simulink model "gm_sampleModel1507_5_sub"  (R2023a)
settings: Solver=VariableStepAuto  StartTime=0.0  StopTime=10.0  RelTol=1e-3
libraries: simulink x3
settings Model: Creator=user1  LastModifiedBy=user1
settings OptimizationCC: BlockReduction=off  ConditionallyExecuteInputs=off
settings DebuggingCC: InheritedTsInSrcMsg=none

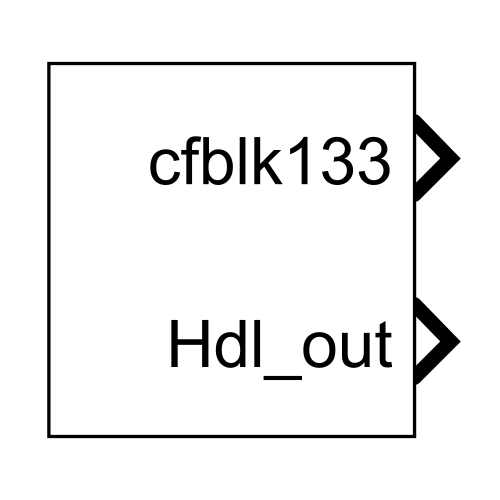
[thumbnail: Simulink's stored preview of the top-level diagram]
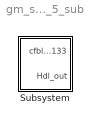
== system gm_sampleModel1507_5_sub ==
  Subsystem : Subsystem

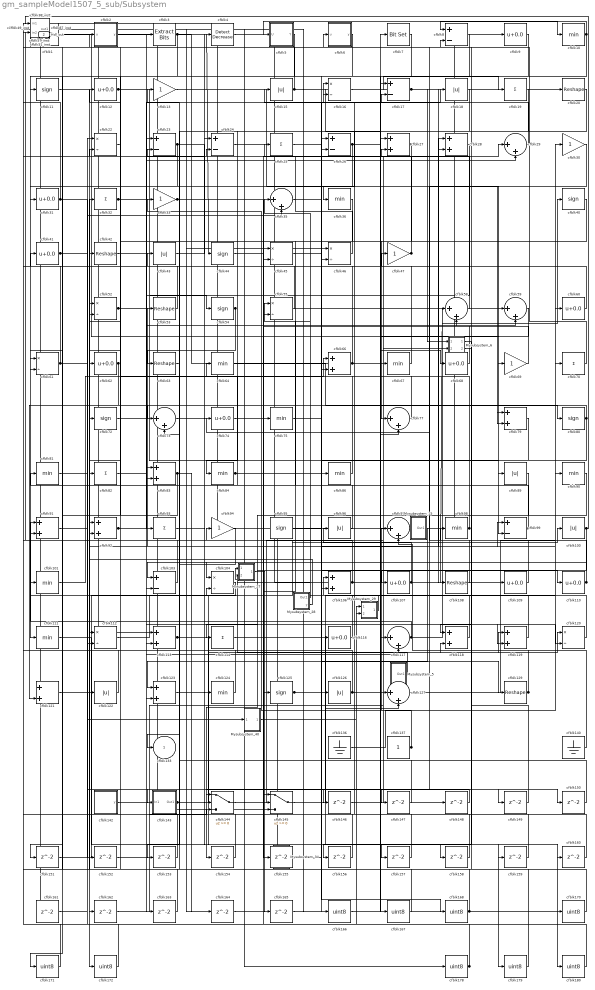
== system gm_sampleModel1507_5_sub/Subsystem ==
  Mysubsystem_15 : Subsystem
  Mysubsystem_27 : Subsystem
  Mysubsystem_28 : Subsystem
  Mysubsystem_29 : Subsystem
  Mysubsystem_34 : Subsystem
  Mysubsystem_40 : Subsystem
  Mysubsystem_5 : Subsystem
  Mysubsystem_6 : Subsystem
  cfblk1 : Logic  AllPortsSameDT=off  OutDataTypeStr=boolean
  cfblk{10,36,64,67,75,81,84,86,90,98,101,111,124} (13 alike) : MinMax  OutDataTypeStr=uint8
  cfblk{15,18,43,89,96,100,122,126} (8 alike) : Abs  OutDataTypeStr=uint8  SaturateOnIntegerOverflow=off
  cfblk102_inst : Subsystem
  cfblk{8,17,23..24,26,99,103} (7 alike) : Sum  Inputs=+-  OutDataTypeStr=uint8
  cfblk{16,22,45..46,52,55,61,104,112,120} (10 alike) : Product  Inputs=*/  OutDataTypeStr=uint8  RndMeth=Zero  SaturateOnIntegerOverflow=on
  cfblk{27..28,66,79,83,91..92,106,113,118..119,121,123} (13 alike) : Sum  OutDataTypeStr=uint8
  cfblk{9,12,31,41,60,62,68,74,107,109..110,116} (12 alike) : Bias  Bias=0.0  SaturateOnIntegerOverflow=off
  cfblk{20,42,53,63,108,129} (6 alike) : Reshape
  cfblk{11,40,44,54,72,80,95,125} (8 alike) : Signum
  cfblk{19,25,32,70,82,93,114} (7 alike) : Sum  Inputs=+  OutDataTypeStr=uint8
  cfblk{29,35,58..59,73,77,97,117,127} (9 alike) : Sum  Inputs=|++  OutDataTypeStr=uint8
  cfblk128_inst : Subsystem
  cfblk{13,30,33,47,69,94} (6 alike) : Gain  OutDataTypeStr=uint8
  cfblk136 : Ground
  cfblk137 : Constant  OutDataTypeStr=uint8  SampleTime=-1
  cfblk140 : Ground
  cfblk142 : Subsystem  mask(Counter Limited){uplimit=double(7), tsamp=double(-1)}
      mask prompts: uplimit "Simulink:masks:UpperLimit_MP"; tsamp "Simulink:masks:SampleTime_MP"
      mask help: Simulink:masks:CounterLimited_MD
      mask init:
      | nbits = double(8);
      | tsamp = double(-1);
      | uplimit = double(7);
  cfblk143 : Subsystem
  cfblk144 : Switch  OutDataTypeStr=uint8  SaturateOnIntegerOverflow=off  InputSameDT=off
  cfblk145 : Switch  OutDataTypeStr=uint8  SaturateOnIntegerOverflow=off  InputSameDT=off
  cfblk{146..165} (20 alike) : Delay  SampleTime=1
  cfblk{166..168,170..172,178..180} (9 alike) : DataTypeConversion  OutDataTypeStr=uint8  SaturateOnIntegerOverflow=off  RndMeth=Floor
  cfblk2 : Subsystem  mask(Compare To Zero){relop=<=, OutDataTypeStr=uint8, ZeroCross=on}
      mask prompts: relop "Simulink:masks:Operator_MP"; OutDataTypeStr "Simulink:masks:OutputDataType_MP"; ZeroCross "Simulink:masks:EnableZerocrossingDetection_MP"
      mask help: Simulink:masks:CompareToZero_MD
      mask init:
      | OutDataTypeStr = 'uint8';
      | ZeroCross = 'on';
      | blkName = 'sampleModel1507_5_sub/Subsystem/cfblk2';
      | relop = '<=';
      | setValue = 'fixdt(0, 8)';
      mask TypeOptions relop: == | ~= | < | <= | >= | >
      mask TypeOptions OutDataTypeStr: Simulink:masks:uint8 | Simulink:masks:boolean
      mask Callback ZeroCross: sl('zeroCrossEnable', gcbh);
      mask Display: disp([relop,' 0'])
  cfblk21_inst : Subsystem
  cfblk3 : simulink/Logic and Bit Operations/Extract Bits  bitsToExtract=Upper half  numBits=8  bitIdxRange=[0 7]  outScalingMode=Preserve fixed-point scaling
      settings: LibrarySourceBlock=|
      | hdlsllib/Logic and Bit
      | Operations/Extract Bits
  cfblk34_inst : Subsystem
  cfblk37_inst : Subsystem
  cfblk38_inst : Subsystem
  cfblk4 : simulink/Logic and Bit Operations/Detect Decrease  vinit=0.0  OutDataTypeStr=uint8
      settings: LibrarySourceBlock=|
      | hdlsllib/Logic and Bit
      | Operations/Detect
      | Decrease
  cfblk49_inst : Subsystem
  cfblk5 : Subsystem  mask(Detect Fall Nonpositive){vinit=double(0), InputProcessing=Elements as channels (sample based), OutDataTypeStr=uint8}
      mask prompts: vinit "Simulink:masks:InitialCondition_MP"; InputProcessing "Simulink:masks:InputProcessing_MP"; OutDataTypeStr "Simulink:masks:OutputDataType_MP"
      mask help: Simulink:masks:DetectFallNonpositive_MD
      mask init:
      | InputProcessing = 'Elements as channels (sample based)';
      | OutDataTypeStr = 'uint8';
      | vinit = double(0);
      mask TypeOptions InputProcessing: Simulink:masks:ColumnsAsChannelsFrameBased | Simulink:masks:ElementsAsChannelsSampleBased
      mask TypeOptions OutDataTypeStr: Simulink:masks:uint8 | Simulink:masks:boolean
      mask Display: fprintf('U <= 0\n&  NOT\nU/z <= 0')
  cfblk51_inst : Subsystem
  cfblk57_inst : Subsystem
  cfblk6 : Subsystem  mask(Compare To Zero){relop=<=, OutDataTypeStr=uint8, ZeroCross=on}
      mask prompts: relop "Simulink:masks:Operator_MP"; OutDataTypeStr "Simulink:masks:OutputDataType_MP"; ZeroCross "Simulink:masks:EnableZerocrossingDetection_MP"
      mask help: Simulink:masks:CompareToZero_MD
      mask init:
      | OutDataTypeStr = 'uint8';
      | ZeroCross = 'on';
      | blkName = 'sampleModel1507_5_sub/Subsystem/cfblk6';
      | relop = '<=';
      | setValue = 'fixdt(0, 8)';
      mask TypeOptions relop: == | ~= | < | <= | >= | >
      mask TypeOptions OutDataTypeStr: Simulink:masks:uint8 | Simulink:masks:boolean
      mask Callback ZeroCross: sl('zeroCrossEnable', gcbh);
      mask Display: disp([relop,' 0'])
  cfblk7 : simulink/Logic and Bit Operations/Bit Set  iBit=0
      settings: LibrarySourceBlock=|
      | hdlsllib/Logic and Bit
      | Operations/Bit Set
  cfblk87_inst : Subsystem
  cfblk133 : Outport  OutDataTypeStr=uint8  SampleTime=1  VectorParamsAs1DForOutWhenUnconnected=off
  Hdl_out : Outport  Port=2  OutDataTypeStr=uint8  SampleTime=1
  wires:
  Mysubsystem_15/1(Out1) -> cfblk123/1
  Mysubsystem_27/1(Out1) -> cfblk165/1
  Mysubsystem_28/1(Out1) -> cfblk103/1
  Mysubsystem_28/2(y) -> cfblk172/1
  Mysubsystem_29/1(Out1) -> Mysubsystem_27/1(In1)
  Mysubsystem_34/1(Out1) -> cfblk95/1
  Mysubsystem_40/1(Out1) -> Mysubsystem_29/1(In1)
  Mysubsystem_5/1(Out1) -> Mysubsystem_27/2(In2)
  Mysubsystem_6/1(Out1) -> cfblk156/1
  Mysubsystem_6/2(Out2) -> cfblk157/1
  cfblk1/1 -> cfblk99/2
  cfblk10/1 -> cfblk8/1, cfblk111/1
  cfblk100/1 -> cfblk37_inst/1(in1), cfblk154/1
  cfblk101/1 -> cfblk66/1
  cfblk102_inst/1(out1) -> cfblk166/1, cfblk145/3
  cfblk103/1 -> cfblk102_inst/2(in2)
  cfblk104/1 -> cfblk91/1
  cfblk106/1 -> cfblk87_inst/2(in2), cfblk29/1
  cfblk107/1 -> cfblk96/1, cfblk58/1
  cfblk108/1 -> cfblk74/1
  cfblk109/1 -> cfblk6/1(u)
  cfblk11/1 -> cfblk162/1
  cfblk110/1 -> cfblk37_inst/2(in2), cfblk104/1
  cfblk111/1 -> cfblk150/1
  cfblk112/1 -> cfblk100/1
  cfblk113/1 -> cfblk158/1, Mysubsystem_6/2(In2)
  cfblk114/1 -> cfblk179/1
  cfblk116/1 -> cfblk35/1
  cfblk117/1 -> cfblk40/1, cfblk101/1
  cfblk118/1 -> cfblk94/1
  cfblk119/1 -> cfblk55/1
  cfblk12/1 -> cfblk89/1, cfblk54/1
  cfblk120/1 -> cfblk106/1
  cfblk121/1 -> cfblk159/1
  cfblk122/1 -> cfblk57_inst/1(in1)
  cfblk123/1 -> cfblk120/1
  cfblk124/1 -> cfblk32/1
  cfblk125/1 -> cfblk180/1, cfblk127/2
  cfblk126/1 -> cfblk41/1, cfblk118/2
  cfblk127/1 -> cfblk60/1
  cfblk128_inst/1(out1) -> cfblk113/1, cfblk161/1, cfblk5/1(U)
  cfblk129/1 -> cfblk97/2, cfblk42/1
  cfblk13/1 -> cfblk69/1
  cfblk136/1 -> cfblk90/1
  cfblk137/1 -> cfblk97/1, cfblk33/1
  cfblk140/1 -> cfblk53/1
  cfblk142/1(y) -> cfblk30/1
  cfblk143/1(Out1) -> cfblk77/2, cfblk86/1
  cfblk144/1 -> cfblk26/2
  cfblk145/1 -> cfblk70/1
  cfblk146/1 -> cfblk28/2
  cfblk147/1 -> cfblk26/1
  cfblk148/1 -> cfblk144/1
  cfblk149/1 -> cfblk8/2
  cfblk15/1 -> cfblk57_inst/2(in2), cfblk117/1
  cfblk150/1 -> cfblk23/2
  cfblk151/1 -> cfblk104/2
  cfblk152/1 -> cfblk144/3
  cfblk153/1 -> cfblk92/2
  cfblk154/1 -> cfblk52/1
  cfblk155/1 -> cfblk99/1
  cfblk156/1 -> cfblk1/1
  cfblk157/1 -> cfblk112/1
  cfblk158/1 -> cfblk16/1
  cfblk159/1 -> cfblk91/2
  cfblk16/1 -> cfblk19/1
  cfblk160/1 -> cfblk83/1
  cfblk161/1 -> cfblk35/2
  cfblk162/1 -> cfblk17/1
  cfblk163/1 -> cfblk1/2
  cfblk164/1 -> cfblk27/2
  cfblk165/1 -> cfblk119/1
  cfblk166/1 -> cfblk7/1
  cfblk167/1 -> cfblk43/1
  cfblk168/1 -> cfblk122/1, cfblk22/2
  cfblk17/1 -> cfblk108/1, Mysubsystem_6/1(In1)
  cfblk170/1 -> cfblk98/1
  cfblk171/1 -> cfblk34_inst/1(in1)
  cfblk172/1 -> cfblk34_inst/2(in2)
  cfblk178/1 -> cfblk145/2, cfblk22/1, Mysubsystem_29/2(In2)
  cfblk179/1 -> cfblk51_inst/1(in1)
  cfblk18/1 -> cfblk84/1
  cfblk180/1 -> cfblk51_inst/2(in2)
  cfblk19/1 -> cfblk63/1
  cfblk2/1(y) -> cfblk163/1
  cfblk20/1 -> cfblk36/1
  cfblk21_inst/1(out1) -> cfblk20/1, cfblk75/1
  cfblk22/1 -> cfblk92/1
  cfblk23/1 -> cfblk144/2, cfblk61/2
  cfblk24/1 -> cfblk79/1
  cfblk25/1 -> cfblk129/1
  cfblk26/1 -> cfblk79/2, cfblk68/1, cfblk103/2
  cfblk27/1 -> cfblk77/1, cfblk125/1, cfblk133/1
  cfblk28/1 -> cfblk83/2
  cfblk29/1 -> cfblk15/1
  cfblk3/1 -> cfblk44/1, cfblk82/1
  cfblk30/1 -> cfblk107/1
  cfblk31/1 -> cfblk49_inst/2(in2), cfblk149/1
  cfblk32/1 -> cfblk29/2, cfblk120/2
  cfblk33/1 -> cfblk73/1, cfblk45/2
  cfblk34_inst/1(out1) -> cfblk170/1
  cfblk35/1 -> cfblk110/1
  cfblk36/1 -> cfblk62/1
  cfblk37_inst/1(out1) -> cfblk38_inst/2(in2), cfblk3/1, cfblk93/1
  cfblk38_inst/1(out1) -> cfblk121/1, cfblk46/1
  cfblk4/1 -> cfblk10/1
  cfblk40/1 -> cfblk46/2
  cfblk41/1 -> cfblk152/1, cfblk151/1
  cfblk42/1 -> cfblk59/2
  cfblk43/1 -> cfblk4/1
  cfblk44/1 -> cfblk155/1
  cfblk45/1 -> cfblk17/2
  cfblk46/1 -> cfblk24/2
  cfblk47/1 -> cfblk21_inst/1(in1), cfblk128_inst/2(in2)
  cfblk49_inst/1(out1) -> cfblk148/1
  cfblk5/1(Y) -> cfblk11/1
  cfblk51_inst/1(out1) -> cfblk178/1
  cfblk52/1 -> cfblk58/2, cfblk24/1
  cfblk53/1 -> cfblk128_inst/1(in1)
  cfblk54/1 -> cfblk73/2, cfblk123/2
  cfblk55/1 -> cfblk23/1
  cfblk57_inst/1(out1) -> cfblk109/1
  cfblk58/1 -> cfblk25/1
  cfblk59/1 -> cfblk67/1
  cfblk6/1(y) -> cfblk61/1
  cfblk60/1 -> cfblk47/1
  cfblk61/1 -> cfblk87_inst/1(in1), Mysubsystem_40/1(In1)
  cfblk62/1 -> cfblk121/2, cfblk112/2
  cfblk63/1 -> cfblk13/1
  cfblk64/1 -> cfblk80/1
  cfblk66/1 -> cfblk38_inst/1(in1), cfblk127/1, Hdl_out/1
  cfblk67/1 -> cfblk49_inst/1(in1)
  cfblk68/1 -> cfblk27/1
  cfblk69/1 -> cfblk45/1
  cfblk7/1 -> cfblk167/1
  cfblk70/1 -> cfblk21_inst/2(in2)
  cfblk72/1 -> cfblk119/2
  cfblk73/1 -> cfblk124/1
  cfblk74/1 -> cfblk116/1
  cfblk75/1 -> cfblk126/1
  cfblk77/1 -> cfblk2/1(u)
  cfblk79/1 -> cfblk147/1
  cfblk8/1 -> cfblk31/1
  cfblk80/1 -> cfblk72/1, cfblk106/2
  cfblk81/1 -> cfblk146/1
  cfblk82/1 -> cfblk113/2
  cfblk83/1 -> cfblk171/1, cfblk164/1
  cfblk84/1 -> cfblk28/1, cfblk145/1
  cfblk86/1 -> cfblk52/2
  cfblk87_inst/1(out1) -> cfblk59/1
  cfblk89/1 -> cfblk114/1
  cfblk9/1 -> cfblk66/2
  cfblk90/1 -> cfblk118/1
  cfblk91/1 -> cfblk143/1(In1)
  cfblk92/1 -> cfblk18/1, cfblk117/2
  cfblk93/1 -> cfblk160/1
  cfblk94/1 -> cfblk153/1
  cfblk95/1 -> cfblk168/1
  cfblk96/1 -> cfblk12/1
  cfblk97/1 -> cfblk9/1, cfblk102_inst/1(in1)
  cfblk98/1 -> cfblk16/2, cfblk81/1
  cfblk99/1 -> cfblk55/2, cfblk64/1

== system gm_sampleModel1507_5_sub/Subsystem/Mysubsystem_15 ==
  cfblk139 : Subsystem  mask(Counter Free-Running){NumBits=double(16), tsamp=double(-1)}
      mask prompts: NumBits "Simulink:masks:NumberOfBits_MP"; tsamp "Simulink:masks:SampleTime_MP"
      mask help: Simulink:masks:CounterFreeRunning_MD
  cfblk65 : Signum
  cfblk88 : Gain
  Out1 : Outport  SampleTime=1
  wires:
  cfblk139/1(y) -> cfblk65/1
  cfblk65/1 -> cfblk88/1
  cfblk88/1 -> Out1/1

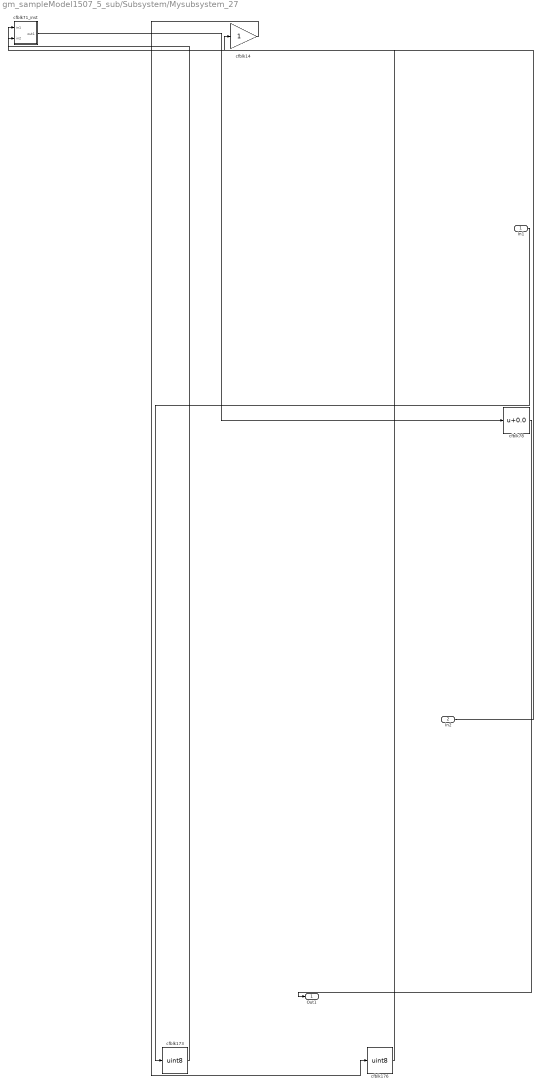
== system gm_sampleModel1507_5_sub/Subsystem/Mysubsystem_27 ==
  In1 : Inport  OutDataTypeStr=uint8  PortDimensions=1  SampleTime=1
  In2 : Inport  Port=2  OutDataTypeStr=uint8  PortDimensions=1  SampleTime=1
  cfblk14 : Gain
  cfblk173 : DataTypeConversion  OutDataTypeStr=uint8  SaturateOnIntegerOverflow=off  RndMeth=Floor
  cfblk176 : DataTypeConversion  OutDataTypeStr=uint8  SaturateOnIntegerOverflow=off  RndMeth=Floor
  cfblk71_inst : Subsystem
  cfblk78 : Bias  Bias=0.0  SaturateOnIntegerOverflow=off
  Out1 : Outport  SampleTime=1
  wires:
  In1/1 -> cfblk173/1
  In2/1 -> cfblk14/1
  cfblk14/1 -> cfblk176/1
  cfblk173/1 -> cfblk71_inst/1(in1)
  cfblk176/1 -> cfblk71_inst/2(in2)
  cfblk71_inst/1(out1) -> cfblk78/1
  cfblk78/1 -> Out1/1

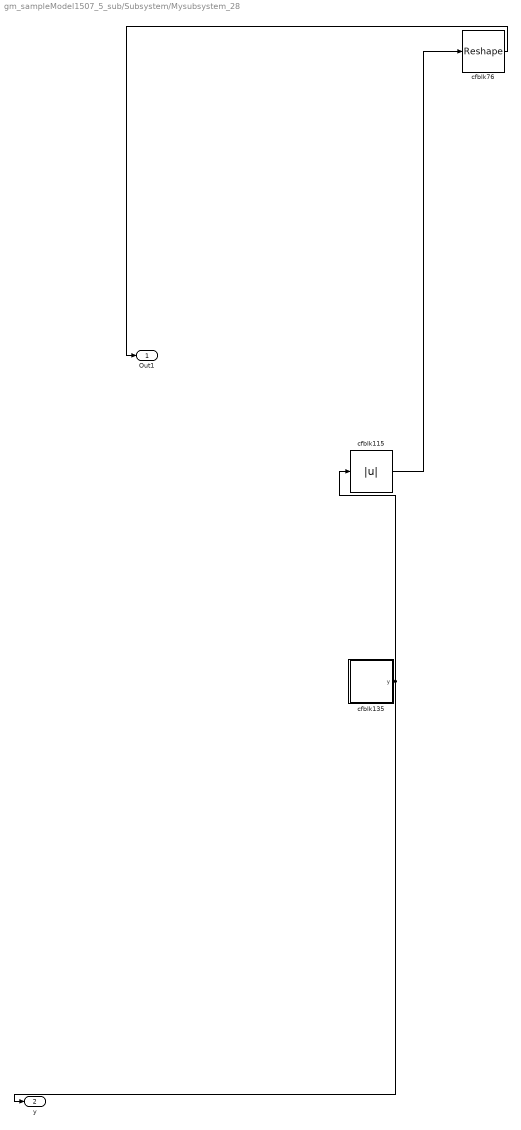
== system gm_sampleModel1507_5_sub/Subsystem/Mysubsystem_28 ==
  cfblk115 : Abs  SaturateOnIntegerOverflow=off
  cfblk135 : Subsystem  mask(Counter Free-Running){NumBits=double(16), tsamp=double(-1)}
      mask prompts: NumBits "Simulink:masks:NumberOfBits_MP"; tsamp "Simulink:masks:SampleTime_MP"
      mask help: Simulink:masks:CounterFreeRunning_MD
  cfblk76 : Reshape
  Out1 : Outport  SampleTime=1
  y : Outport  Port=2  SampleTime=1
  wires:
  cfblk115/1 -> cfblk76/1
  cfblk135/1(y) -> cfblk115/1, y/1
  cfblk76/1 -> Out1/1

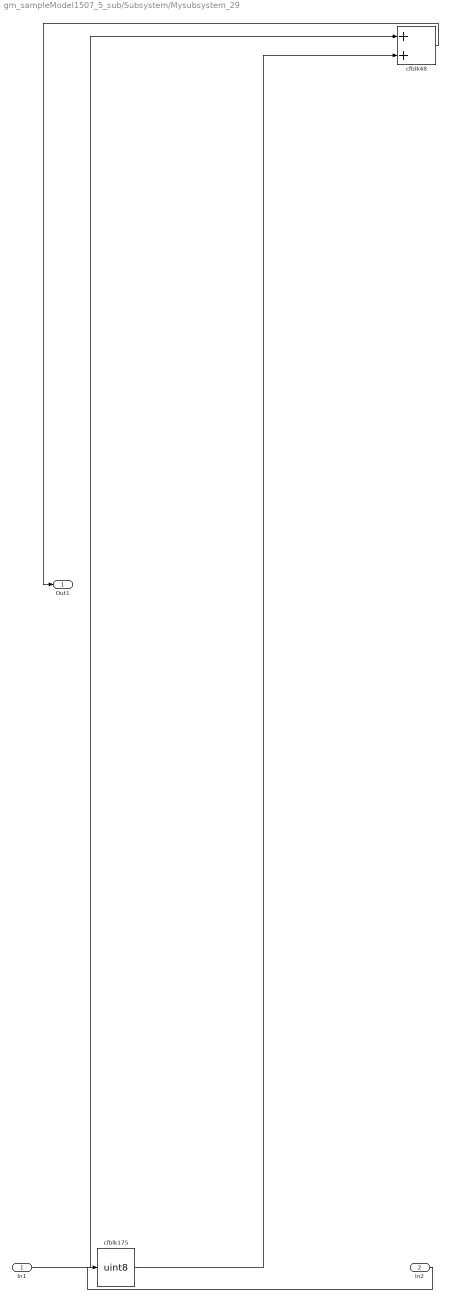
== system gm_sampleModel1507_5_sub/Subsystem/Mysubsystem_29 ==
  In1 : Inport  OutDataTypeStr=uint8  PortDimensions=1  SampleTime=1
  In2 : Inport  Port=2  OutDataTypeStr=uint8  PortDimensions=1  SampleTime=1
  cfblk175 : DataTypeConversion  OutDataTypeStr=uint8  SaturateOnIntegerOverflow=off  RndMeth=Floor
  cfblk48 : Sum
  Out1 : Outport  SampleTime=1
  wires:
  In1/1 -> cfblk48/1
  In2/1 -> cfblk175/1
  cfblk175/1 -> cfblk48/2
  cfblk48/1 -> Out1/1

== system gm_sampleModel1507_5_sub/Subsystem/Mysubsystem_34 ==
  cfblk141 : Subsystem  mask(Counter Free-Running){NumBits=double(16), tsamp=double(-1)}
      mask prompts: NumBits "Simulink:masks:NumberOfBits_MP"; tsamp "Simulink:masks:SampleTime_MP"
      mask help: Simulink:masks:CounterFreeRunning_MD
  cfblk169 : DataTypeConversion  OutDataTypeStr=uint8  SaturateOnIntegerOverflow=off  RndMeth=Floor
  Out1 : Outport  SampleTime=1
  wires:
  cfblk141/1(y) -> cfblk169/1
  cfblk169/1 -> Out1/1

== system gm_sampleModel1507_5_sub/Subsystem/Mysubsystem_40 ==
  In1 : Inport  OutDataTypeStr=uint8  PortDimensions=1  SampleTime=1
  cfblk174 : DataTypeConversion  OutDataTypeStr=uint8  SaturateOnIntegerOverflow=off  RndMeth=Floor
  cfblk85 : Abs  SaturateOnIntegerOverflow=off
  Out1 : Outport  SampleTime=1
  wires:
  In1/1 -> cfblk85/1
  cfblk174/1 -> Out1/1
  cfblk85/1 -> cfblk174/1

== system gm_sampleModel1507_5_sub/Subsystem/Mysubsystem_5 ==
  cfblk138 : Subsystem  mask(Counter Limited){uplimit=double(7), tsamp=double(-1)}
      mask prompts: uplimit "Simulink:masks:UpperLimit_MP"; tsamp "Simulink:masks:SampleTime_MP"
      mask help: Simulink:masks:CounterLimited_MD
      mask init:
      | nbits = double(8);
      | tsamp = double(-1);
      | uplimit = double(7);
  cfblk177 : DataTypeConversion  OutDataTypeStr=uint8  SaturateOnIntegerOverflow=off  RndMeth=Floor
  cfblk56 : Abs  SaturateOnIntegerOverflow=off
  Out1 : Outport  SampleTime=1
  wires:
  cfblk138/1(y) -> cfblk56/1
  cfblk177/1 -> Out1/1
  cfblk56/1 -> cfblk177/1

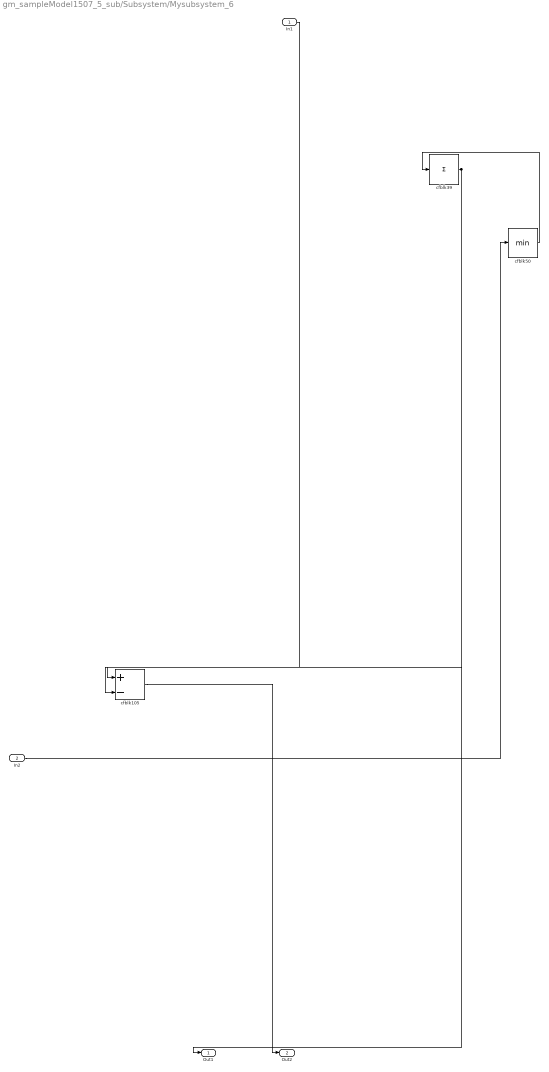
== system gm_sampleModel1507_5_sub/Subsystem/Mysubsystem_6 ==
  In1 : Inport  OutDataTypeStr=uint8  PortDimensions=1  SampleTime=1
  In2 : Inport  Port=2  OutDataTypeStr=uint8  PortDimensions=1  SampleTime=1
  cfblk105 : Sum  Inputs=+-
  cfblk39 : Sum  Inputs=+
  cfblk50 : MinMax
  Out1 : Outport  SampleTime=1
  Out2 : Outport  Port=2  SampleTime=1
  wires:
  In1/1 -> cfblk105/1
  In2/1 -> cfblk50/1
  cfblk105/1 -> Out2/1
  cfblk39/1 -> cfblk105/2, Out1/1
  cfblk50/1 -> cfblk39/1

== system gm_sampleModel1507_5_sub/Subsystem/cfblk102_inst ==
  in1 : Inport  OutDataTypeStr=uint8  SampleTime=1
  in2 : Inport  Port=2  OutDataTypeStr=uint8  SampleTime=1
  mul_cfblk102_dotp_mulcomp : Product  Inputs=**  OutDataTypeStr=uint8  SampleTime=1
  out1 : Outport  OutDataTypeStr=uint8  SampleTime=1
  wires:
  in1/1 -> mul_cfblk102_dotp_mulcomp/1
  in2/1 -> mul_cfblk102_dotp_mulcomp/2
  mul_cfblk102_dotp_mulcomp/1 -> out1/1

== system gm_sampleModel1507_5_sub/Subsystem/cfblk128_inst ==
  in1 : Inport  OutDataTypeStr=uint8  SampleTime=1
  in2 : Inport  Port=2  OutDataTypeStr=uint8  SampleTime=1
  mul_cfblk128_dotp_mulcomp : Product  Inputs=**  OutDataTypeStr=uint8  SampleTime=1
  out1 : Outport  OutDataTypeStr=uint8  SampleTime=1
  wires:
  in1/1 -> mul_cfblk128_dotp_mulcomp/1
  in2/1 -> mul_cfblk128_dotp_mulcomp/2
  mul_cfblk128_dotp_mulcomp/1 -> out1/1

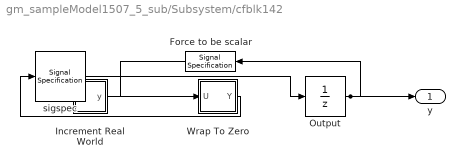
== system gm_sampleModel1507_5_sub/Subsystem/cfblk142 ==
  Force to be scalar : SignalSpecification  DisableCoverage=on  Dimensions=1
  Increment Real World : Subsystem  mask(Real World Value Increment){}
      mask help: Simulink:masks:RealWorldValueIncrement_MD
      mask Display: disp('V++')
  Output : UnitDelay  InitialCondition=0.0  SampleTime=tsamp  HasFrameUpgradeWarning=on
  Wrap To Zero : Subsystem  mask(Wrap To Zero){Threshold=double(7)}
      mask prompts: Threshold "Simulink:masks:Threshold_MP"
      mask help: Simulink:masks:WrapToZero_MD
  sigspec : SignalSpecification  OutDataTypeStr=uint8  Dimensions=1
  y : Outport  SampleTime=1
  wires:
  Force to be scalar/1 -> Increment Real World/1(u)
  Increment Real World/1(y) -> Wrap To Zero/1(U)
  Output/1 -> Force to be scalar/1, y/1
  Wrap To Zero/1(Y) -> sigspec/1
  sigspec/1 -> Output/1

== system gm_sampleModel1507_5_sub/Subsystem/cfblk143 ==
  In1 : Inport  OutDataTypeStr=uint8  PortDimensions=1  SampleTime=1
  Out1 : Outport  SampleTime=1
  wires:
  In1/1 -> Out1/1

== system gm_sampleModel1507_5_sub/Subsystem/cfblk2 ==
  u : Inport  OutDataTypeStr=uint8  SampleTime=1
  Compare : RelationalOperator  Operator=<=  OutDataTypeStr=fixdt(0, 8)
  Constant : Constant  DisableCoverage=on  Value=0  OutDataTypeStr=Inherit: Inherit via back propagation  SampleTime=-1  PreserveConstantTs=on
  y : Outport  SampleTime=1
  wires:
  u/1 -> Compare/1
  Compare/1 -> y/1
  Constant/1 -> Compare/2

== system gm_sampleModel1507_5_sub/Subsystem/cfblk21_inst ==
  in1 : Inport  OutDataTypeStr=uint8  SampleTime=1
  in2 : Inport  Port=2  OutDataTypeStr=uint8  SampleTime=1
  mul_cfblk21_dotp_mulcomp : Product  Inputs=**  OutDataTypeStr=uint8  SampleTime=1
  out1 : Outport  OutDataTypeStr=uint8  SampleTime=1
  wires:
  in1/1 -> mul_cfblk21_dotp_mulcomp/1
  in2/1 -> mul_cfblk21_dotp_mulcomp/2
  mul_cfblk21_dotp_mulcomp/1 -> out1/1

== system gm_sampleModel1507_5_sub/Subsystem/cfblk34_inst ==
  in1 : Inport  OutDataTypeStr=uint8  SampleTime=1
  in2 : Inport  Port=2  OutDataTypeStr=uint8  SampleTime=1
  mul_cfblk34_dotp_mulcomp : Product  Inputs=**  OutDataTypeStr=uint8  SampleTime=1
  out1 : Outport  OutDataTypeStr=uint8  SampleTime=1
  wires:
  in1/1 -> mul_cfblk34_dotp_mulcomp/1
  in2/1 -> mul_cfblk34_dotp_mulcomp/2
  mul_cfblk34_dotp_mulcomp/1 -> out1/1

== system gm_sampleModel1507_5_sub/Subsystem/cfblk37_inst ==
  in1 : Inport  OutDataTypeStr=uint8  SampleTime=1
  in2 : Inport  Port=2  OutDataTypeStr=uint8  SampleTime=1
  mul_cfblk37_dotp_mulcomp : Product  Inputs=**  OutDataTypeStr=uint8  SampleTime=1
  out1 : Outport  OutDataTypeStr=uint8  SampleTime=1
  wires:
  in1/1 -> mul_cfblk37_dotp_mulcomp/1
  in2/1 -> mul_cfblk37_dotp_mulcomp/2
  mul_cfblk37_dotp_mulcomp/1 -> out1/1

== system gm_sampleModel1507_5_sub/Subsystem/cfblk38_inst ==
  in1 : Inport  OutDataTypeStr=uint8  SampleTime=1
  in2 : Inport  Port=2  OutDataTypeStr=uint8  SampleTime=1
  mul_cfblk38_dotp_mulcomp : Product  Inputs=**  OutDataTypeStr=uint8  SampleTime=1
  out1 : Outport  OutDataTypeStr=uint8  SampleTime=1
  wires:
  in1/1 -> mul_cfblk38_dotp_mulcomp/1
  in2/1 -> mul_cfblk38_dotp_mulcomp/2
  mul_cfblk38_dotp_mulcomp/1 -> out1/1

== system gm_sampleModel1507_5_sub/Subsystem/cfblk49_inst ==
  in1 : Inport  OutDataTypeStr=uint8  SampleTime=1
  in2 : Inport  Port=2  OutDataTypeStr=uint8  SampleTime=1
  mul_cfblk49_dotp_mulcomp : Product  Inputs=**  OutDataTypeStr=uint8  SampleTime=1
  out1 : Outport  OutDataTypeStr=uint8  SampleTime=1
  wires:
  in1/1 -> mul_cfblk49_dotp_mulcomp/1
  in2/1 -> mul_cfblk49_dotp_mulcomp/2
  mul_cfblk49_dotp_mulcomp/1 -> out1/1

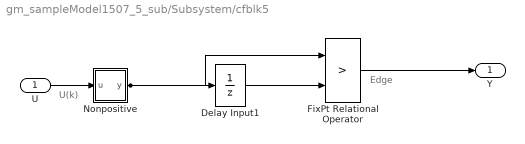
== system gm_sampleModel1507_5_sub/Subsystem/cfblk5 ==
  note: U(k)
  note: Edge
  U : Inport  OutDataTypeStr=uint8  SampleTime=1
  Delay Input1 : UnitDelay  Description=Store in Global RAM  DisableCoverage=on  InitialCondition=vinit  SampleTime=-1  HasFrameUpgradeWarning=on
  FixPt Relational Operator : RelationalOperator  Operator=>  OutDataTypeStr=fixdt(0, 8)  ZeroCross=off  InputSameDT=off
  Nonpositive : Subsystem  mask(Compare To Zero){relop=<=, OutDataTypeStr=boolean, ZeroCross=off}
      mask prompts: relop "Simulink:masks:Operator_MP"; OutDataTypeStr "Simulink:masks:OutputDataType_MP"; ZeroCross "Simulink:masks:EnableZerocrossingDetection_MP"
      mask help: Simulink:masks:CompareToZero_MD
      mask init:
      | OutDataTypeStr = 'boolean';
      | ZeroCross = 'off';
      | blkName = 'sampleModel1507_5_sub/Subsystem/cfblk5/Nonpositive';
      | relop = '<=';
      | setValue = 'boolean';
      mask TypeOptions relop: == | ~= | < | <= | >= | >
      mask TypeOptions OutDataTypeStr: Simulink:masks:uint8 | Simulink:masks:boolean
      mask Callback ZeroCross: sl('zeroCrossEnable', gcbh);
      mask Display: disp([relop,' 0'])
  Y : Outport  SampleTime=1
  wires:
  U/1 -> Nonpositive/1(u)
  Delay Input1/1 -> FixPt Relational Operator/2
  FixPt Relational Operator/1 -> Y/1
  Nonpositive/1(y) -> FixPt Relational Operator/1, Delay Input1/1

== system gm_sampleModel1507_5_sub/Subsystem/cfblk51_inst ==
  in1 : Inport  OutDataTypeStr=uint8  SampleTime=1
  in2 : Inport  Port=2  OutDataTypeStr=uint8  SampleTime=1
  mul_cfblk51_dotp_mulcomp : Product  Inputs=**  OutDataTypeStr=uint8  SampleTime=1
  out1 : Outport  OutDataTypeStr=uint8  SampleTime=1
  wires:
  in1/1 -> mul_cfblk51_dotp_mulcomp/1
  in2/1 -> mul_cfblk51_dotp_mulcomp/2
  mul_cfblk51_dotp_mulcomp/1 -> out1/1

== system gm_sampleModel1507_5_sub/Subsystem/cfblk57_inst ==
  in1 : Inport  OutDataTypeStr=uint8  SampleTime=1
  in2 : Inport  Port=2  OutDataTypeStr=uint8  SampleTime=1
  mul_cfblk57_dotp_mulcomp : Product  Inputs=**  OutDataTypeStr=uint8  SampleTime=1
  out1 : Outport  OutDataTypeStr=uint8  SampleTime=1
  wires:
  in1/1 -> mul_cfblk57_dotp_mulcomp/1
  in2/1 -> mul_cfblk57_dotp_mulcomp/2
  mul_cfblk57_dotp_mulcomp/1 -> out1/1

== system gm_sampleModel1507_5_sub/Subsystem/cfblk6 ==
  u : Inport  OutDataTypeStr=uint8  SampleTime=1
  Compare : RelationalOperator  Operator=<=  OutDataTypeStr=fixdt(0, 8)
  Constant : Constant  DisableCoverage=on  Value=0  OutDataTypeStr=Inherit: Inherit via back propagation  SampleTime=-1  PreserveConstantTs=on
  y : Outport  SampleTime=1
  wires:
  u/1 -> Compare/1
  Compare/1 -> y/1
  Constant/1 -> Compare/2

== system gm_sampleModel1507_5_sub/Subsystem/cfblk87_inst ==
  in1 : Inport  OutDataTypeStr=uint8  SampleTime=1
  in2 : Inport  Port=2  OutDataTypeStr=uint8  SampleTime=1
  mul_cfblk87_dotp_mulcomp : Product  Inputs=**  OutDataTypeStr=uint8  SampleTime=1
  out1 : Outport  OutDataTypeStr=uint8  SampleTime=1
  wires:
  in1/1 -> mul_cfblk87_dotp_mulcomp/1
  in2/1 -> mul_cfblk87_dotp_mulcomp/2
  mul_cfblk87_dotp_mulcomp/1 -> out1/1

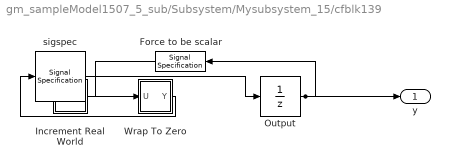
== system gm_sampleModel1507_5_sub/Subsystem/Mysubsystem_15/cfblk139 ==
  Force to be scalar : SignalSpecification  DisableCoverage=on  Dimensions=1
  Increment Real World : Subsystem  mask(Real World Value Increment){}
      mask help: Simulink:masks:RealWorldValueIncrement_MD
      mask Display: disp('V++')
  Output : UnitDelay  InitialCondition=0.0  SampleTime=tsamp  HasFrameUpgradeWarning=on
  Wrap To Zero : Subsystem  mask(Wrap To Zero){Threshold=double(65535)}
      mask prompts: Threshold "Simulink:masks:Threshold_MP"
      mask help: Simulink:masks:WrapToZero_MD
  sigspec : SignalSpecification  OutDataTypeStr=uint16  Dimensions=1
  y : Outport  SampleTime=1
  wires:
  Force to be scalar/1 -> Increment Real World/1(u)
  Increment Real World/1(y) -> Wrap To Zero/1(U)
  Output/1 -> Force to be scalar/1, y/1
  Wrap To Zero/1(Y) -> sigspec/1
  sigspec/1 -> Output/1

== system gm_sampleModel1507_5_sub/Subsystem/Mysubsystem_27/cfblk71_inst ==
  in1 : Inport  OutDataTypeStr=uint8  SampleTime=1
  in2 : Inport  Port=2  OutDataTypeStr=uint8  SampleTime=1
  mul_cfblk71_dotp_mulcomp : Product  Inputs=**  OutDataTypeStr=uint16  SampleTime=1
  out1 : Outport  OutDataTypeStr=uint16  SampleTime=1
  wires:
  in1/1 -> mul_cfblk71_dotp_mulcomp/1
  in2/1 -> mul_cfblk71_dotp_mulcomp/2
  mul_cfblk71_dotp_mulcomp/1 -> out1/1

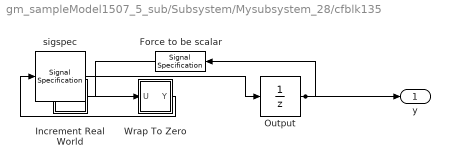
== system gm_sampleModel1507_5_sub/Subsystem/Mysubsystem_28/cfblk135 ==
  Force to be scalar : SignalSpecification  DisableCoverage=on  Dimensions=1
  Increment Real World : Subsystem  mask(Real World Value Increment){}
      mask help: Simulink:masks:RealWorldValueIncrement_MD
      mask Display: disp('V++')
  Output : UnitDelay  InitialCondition=0.0  SampleTime=tsamp  HasFrameUpgradeWarning=on
  Wrap To Zero : Subsystem  mask(Wrap To Zero){Threshold=double(65535)}
      mask prompts: Threshold "Simulink:masks:Threshold_MP"
      mask help: Simulink:masks:WrapToZero_MD
  sigspec : SignalSpecification  OutDataTypeStr=uint16  Dimensions=1
  y : Outport  SampleTime=1
  wires:
  Force to be scalar/1 -> Increment Real World/1(u)
  Increment Real World/1(y) -> Wrap To Zero/1(U)
  Output/1 -> Force to be scalar/1, y/1
  Wrap To Zero/1(Y) -> sigspec/1
  sigspec/1 -> Output/1

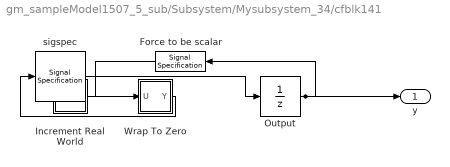
== system gm_sampleModel1507_5_sub/Subsystem/Mysubsystem_34/cfblk141 ==
  Force to be scalar : SignalSpecification  DisableCoverage=on  Dimensions=1
  Increment Real World : Subsystem  mask(Real World Value Increment){}
      mask help: Simulink:masks:RealWorldValueIncrement_MD
      mask Display: disp('V++')
  Output : UnitDelay  InitialCondition=0.0  SampleTime=tsamp  HasFrameUpgradeWarning=on
  Wrap To Zero : Subsystem  mask(Wrap To Zero){Threshold=double(65535)}
      mask prompts: Threshold "Simulink:masks:Threshold_MP"
      mask help: Simulink:masks:WrapToZero_MD
  sigspec : SignalSpecification  OutDataTypeStr=uint16  Dimensions=1
  y : Outport  SampleTime=1
  wires:
  Force to be scalar/1 -> Increment Real World/1(u)
  Increment Real World/1(y) -> Wrap To Zero/1(U)
  Output/1 -> Force to be scalar/1, y/1
  Wrap To Zero/1(Y) -> sigspec/1
  sigspec/1 -> Output/1

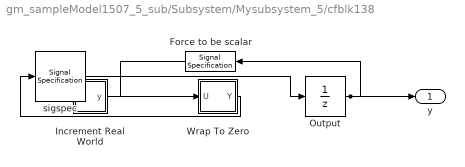
== system gm_sampleModel1507_5_sub/Subsystem/Mysubsystem_5/cfblk138 ==
  Force to be scalar : SignalSpecification  DisableCoverage=on  Dimensions=1
  Increment Real World : Subsystem  mask(Real World Value Increment){}
      mask help: Simulink:masks:RealWorldValueIncrement_MD
      mask Display: disp('V++')
  Output : UnitDelay  InitialCondition=0.0  SampleTime=tsamp  HasFrameUpgradeWarning=on
  Wrap To Zero : Subsystem  mask(Wrap To Zero){Threshold=double(7)}
      mask prompts: Threshold "Simulink:masks:Threshold_MP"
      mask help: Simulink:masks:WrapToZero_MD
  sigspec : SignalSpecification  OutDataTypeStr=uint8  Dimensions=1
  y : Outport  SampleTime=1
  wires:
  Force to be scalar/1 -> Increment Real World/1(u)
  Increment Real World/1(y) -> Wrap To Zero/1(U)
  Output/1 -> Force to be scalar/1, y/1
  Wrap To Zero/1(Y) -> sigspec/1
  sigspec/1 -> Output/1

== system gm_sampleModel1507_5_sub/Subsystem/cfblk142/Increment Real World ==
  u : Inport  OutDataTypeStr=uint8  SampleTime=1
  FixPt Constant : Constant  DisableCoverage=on  OutDataTypeStr=Inherit: Inherit via back propagation  SampleTime=-1
  FixPt Data Type Duplicate : DataTypeDuplicate  DisableCoverage=on  NumInputPorts=3
  FixPt Sum1 : Sum  InputSameDT=on  OutDataTypeStr=Inherit: Inherit via back propagation  LockScale=on
  y : Outport  SampleTime=1
  wires:
  u/1 -> FixPt Sum1/1, FixPt Data Type Duplicate/2
  FixPt Constant/1 -> FixPt Sum1/2, FixPt Data Type Duplicate/3
  FixPt Sum1/1 -> FixPt Data Type Duplicate/1, y/1

== system gm_sampleModel1507_5_sub/Subsystem/cfblk142/Wrap To Zero ==
  note: U(k)
  U : Inport  OutDataTypeStr=uint8  SampleTime=1
  Constant : Constant  DisableCoverage=on  Value=0  OutDataTypeStr=Inherit: Inherit via back propagation  SampleTime=-1
  FixPt Data Type Duplicate1 : DataTypeDuplicate  DisableCoverage=on  NumInputPorts=3
  FixPt Switch : Switch  Criteria=u2 > Threshold  Threshold=Threshold  OutDataTypeStr=Inherit: Inherit via back propagation  ZeroCross=off  SaturateOnIntegerOverflow=off  InputSameDT=off
  Y : Outport  SampleTime=1
  wires:
  U/1 -> FixPt Switch/3, FixPt Switch/2, FixPt Data Type Duplicate1/2
  Constant/1 -> FixPt Switch/1, FixPt Data Type Duplicate1/3
  FixPt Switch/1 -> FixPt Data Type Duplicate1/1, Y/1

== system gm_sampleModel1507_5_sub/Subsystem/cfblk5/Nonpositive ==
  u : Inport  OutDataTypeStr=uint8  SampleTime=1
  Compare : RelationalOperator  Operator=<=  OutDataTypeStr=boolean  ZeroCross=off
  Constant : Constant  DisableCoverage=on  Value=0  OutDataTypeStr=Inherit: Inherit via back propagation  SampleTime=-1  PreserveConstantTs=on
  y : Outport  SampleTime=1
  wires:
  u/1 -> Compare/1
  Compare/1 -> y/1
  Constant/1 -> Compare/2

== system gm_sampleModel1507_5_sub/Subsystem/Mysubsystem_15/cfblk139/Increment Real World ==
  u : Inport  OutDataTypeStr=uint16  SampleTime=1
  FixPt Constant : Constant  DisableCoverage=on  OutDataTypeStr=Inherit: Inherit via back propagation  SampleTime=-1
  FixPt Data Type Duplicate : DataTypeDuplicate  DisableCoverage=on  NumInputPorts=3
  FixPt Sum1 : Sum  InputSameDT=on  OutDataTypeStr=Inherit: Inherit via back propagation  LockScale=on
  y : Outport  SampleTime=1
  wires:
  u/1 -> FixPt Sum1/1, FixPt Data Type Duplicate/2
  FixPt Constant/1 -> FixPt Sum1/2, FixPt Data Type Duplicate/3
  FixPt Sum1/1 -> FixPt Data Type Duplicate/1, y/1

== system gm_sampleModel1507_5_sub/Subsystem/Mysubsystem_15/cfblk139/Wrap To Zero ==
  note: U(k)
  U : Inport  OutDataTypeStr=uint16  SampleTime=1
  Constant : Constant  DisableCoverage=on  Value=0  OutDataTypeStr=Inherit: Inherit via back propagation  SampleTime=-1
  FixPt Data Type Duplicate1 : DataTypeDuplicate  DisableCoverage=on  NumInputPorts=3
  FixPt Switch : Switch  Criteria=u2 > Threshold  Threshold=Threshold  OutDataTypeStr=Inherit: Inherit via back propagation  ZeroCross=off  SaturateOnIntegerOverflow=off  InputSameDT=off
  Y : Outport  SampleTime=1
  wires:
  U/1 -> FixPt Switch/3, FixPt Switch/2, FixPt Data Type Duplicate1/2
  Constant/1 -> FixPt Switch/1, FixPt Data Type Duplicate1/3
  FixPt Switch/1 -> FixPt Data Type Duplicate1/1, Y/1

== system gm_sampleModel1507_5_sub/Subsystem/Mysubsystem_28/cfblk135/Increment Real World ==
  u : Inport  OutDataTypeStr=uint16  SampleTime=1
  FixPt Constant : Constant  DisableCoverage=on  OutDataTypeStr=Inherit: Inherit via back propagation  SampleTime=-1
  FixPt Data Type Duplicate : DataTypeDuplicate  DisableCoverage=on  NumInputPorts=3
  FixPt Sum1 : Sum  InputSameDT=on  OutDataTypeStr=Inherit: Inherit via back propagation  LockScale=on
  y : Outport  SampleTime=1
  wires:
  u/1 -> FixPt Sum1/1, FixPt Data Type Duplicate/2
  FixPt Constant/1 -> FixPt Sum1/2, FixPt Data Type Duplicate/3
  FixPt Sum1/1 -> FixPt Data Type Duplicate/1, y/1

== system gm_sampleModel1507_5_sub/Subsystem/Mysubsystem_28/cfblk135/Wrap To Zero ==
  note: U(k)
  U : Inport  OutDataTypeStr=uint16  SampleTime=1
  Constant : Constant  DisableCoverage=on  Value=0  OutDataTypeStr=Inherit: Inherit via back propagation  SampleTime=-1
  FixPt Data Type Duplicate1 : DataTypeDuplicate  DisableCoverage=on  NumInputPorts=3
  FixPt Switch : Switch  Criteria=u2 > Threshold  Threshold=Threshold  OutDataTypeStr=Inherit: Inherit via back propagation  ZeroCross=off  SaturateOnIntegerOverflow=off  InputSameDT=off
  Y : Outport  SampleTime=1
  wires:
  U/1 -> FixPt Switch/3, FixPt Switch/2, FixPt Data Type Duplicate1/2
  Constant/1 -> FixPt Switch/1, FixPt Data Type Duplicate1/3
  FixPt Switch/1 -> FixPt Data Type Duplicate1/1, Y/1

== system gm_sampleModel1507_5_sub/Subsystem/Mysubsystem_34/cfblk141/Increment Real World ==
  u : Inport  OutDataTypeStr=uint16  SampleTime=1
  FixPt Constant : Constant  DisableCoverage=on  OutDataTypeStr=Inherit: Inherit via back propagation  SampleTime=-1
  FixPt Data Type Duplicate : DataTypeDuplicate  DisableCoverage=on  NumInputPorts=3
  FixPt Sum1 : Sum  InputSameDT=on  OutDataTypeStr=Inherit: Inherit via back propagation  LockScale=on
  y : Outport  SampleTime=1
  wires:
  u/1 -> FixPt Sum1/1, FixPt Data Type Duplicate/2
  FixPt Constant/1 -> FixPt Sum1/2, FixPt Data Type Duplicate/3
  FixPt Sum1/1 -> FixPt Data Type Duplicate/1, y/1

== system gm_sampleModel1507_5_sub/Subsystem/Mysubsystem_34/cfblk141/Wrap To Zero ==
  note: U(k)
  U : Inport  OutDataTypeStr=uint16  SampleTime=1
  Constant : Constant  DisableCoverage=on  Value=0  OutDataTypeStr=Inherit: Inherit via back propagation  SampleTime=-1
  FixPt Data Type Duplicate1 : DataTypeDuplicate  DisableCoverage=on  NumInputPorts=3
  FixPt Switch : Switch  Criteria=u2 > Threshold  Threshold=Threshold  OutDataTypeStr=Inherit: Inherit via back propagation  ZeroCross=off  SaturateOnIntegerOverflow=off  InputSameDT=off
  Y : Outport  SampleTime=1
  wires:
  U/1 -> FixPt Switch/3, FixPt Switch/2, FixPt Data Type Duplicate1/2
  Constant/1 -> FixPt Switch/1, FixPt Data Type Duplicate1/3
  FixPt Switch/1 -> FixPt Data Type Duplicate1/1, Y/1

== system gm_sampleModel1507_5_sub/Subsystem/Mysubsystem_5/cfblk138/Increment Real World ==
  u : Inport  OutDataTypeStr=uint8  SampleTime=1
  FixPt Constant : Constant  DisableCoverage=on  OutDataTypeStr=Inherit: Inherit via back propagation  SampleTime=-1
  FixPt Data Type Duplicate : DataTypeDuplicate  DisableCoverage=on  NumInputPorts=3
  FixPt Sum1 : Sum  InputSameDT=on  OutDataTypeStr=Inherit: Inherit via back propagation  LockScale=on
  y : Outport  SampleTime=1
  wires:
  u/1 -> FixPt Sum1/1, FixPt Data Type Duplicate/2
  FixPt Constant/1 -> FixPt Sum1/2, FixPt Data Type Duplicate/3
  FixPt Sum1/1 -> FixPt Data Type Duplicate/1, y/1

== system gm_sampleModel1507_5_sub/Subsystem/Mysubsystem_5/cfblk138/Wrap To Zero ==
  note: U(k)
  U : Inport  OutDataTypeStr=uint8  SampleTime=1
  Constant : Constant  DisableCoverage=on  Value=0  OutDataTypeStr=Inherit: Inherit via back propagation  SampleTime=-1
  FixPt Data Type Duplicate1 : DataTypeDuplicate  DisableCoverage=on  NumInputPorts=3
  FixPt Switch : Switch  Criteria=u2 > Threshold  Threshold=Threshold  OutDataTypeStr=Inherit: Inherit via back propagation  ZeroCross=off  SaturateOnIntegerOverflow=off  InputSameDT=off
  Y : Outport  SampleTime=1
  wires:
  U/1 -> FixPt Switch/3, FixPt Switch/2, FixPt Data Type Duplicate1/2
  Constant/1 -> FixPt Switch/1, FixPt Data Type Duplicate1/3
  FixPt Switch/1 -> FixPt Data Type Duplicate1/1, Y/1
